simulink model "Angular_Input_Sliding_Mode"  (R2021b)
settings: Solver=VariableStepAuto  StartTime=tspan(1)  StopTime=tspan(2)  RelTol=1e-8
undefined symbols (not defined in the file): b_s1d, b_S2d, BL_gain, K_switch, lambda_1_num, lambda_2_num, r_sim, Tmax, x_0
libraries: slpidlib x2
(part 2 of 2)

== matlab function Angular_Input_Sliding_Mode/Controller x dimension/BL Logic ==
  data: S input; port output; S_BL_value parameter
function port = fcn(S,S_BL_value)

if abs(S) <= S_BL_value

    port = 1; %If we are in the boundary layer, use the boundary layer proportional law

else 
    port = 2; %Outside, use the signum law
end
